simulink model "simscape1"  (R2016b)
settings: Solver=VariableStepAuto  StartTime=0.0  StopTime=3600*3  RelTol=1e-3
libraries: fl_lib x8, nesl_utility x4
settings Model: Creator=Gyulai László  LastModifiedBy=gylaszlo

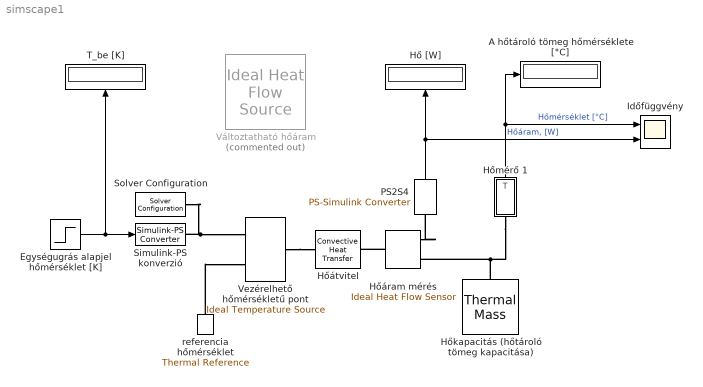
== system simscape1 ==
  A hőtároló tömeg hőmérséklete [°C] : Display
  Egységugrás alapjel hőmérséklet [K] : Step  Before=273  After=293  SampleTime=0
  Hő [W] : Display
  Hőkapacitás (hőtároló tömeg kapacitása) : fl_lib/Thermal/Thermal Elements/Thermal Mass  mass=1.5 kg  sp_heat=840 J/kg/K  T_specify=on  T_priority=High  T=0 degC  Q_specify=off  Q_priority=None  Q=0 J/s
  Hőmérő 1 : Subsystem
  Hőáram mérés : fl_lib/Thermal/Thermal Sensors/Ideal Heat Flow Sensor
  "Hőátvitel " : fl_lib/Thermal/Thermal Elements/Convective Heat Transfer  area=0.125 m^2  heat_tr_coeff=5 W/(m^2 * K)  Q_specify=off  Q_priority=None  Q=0 J/s  T_specify=off  T_priority=None  T=0 K
  Időfüggvény : Scope  NumInputPorts=2
  PS2S4 : nesl_utility/PS-Simulink Converter  PhysicalDomain=network_engine_domain  SubClassName=ps_output  LeftPortType=input  RightPortType=output  PseudoPeriodic=off  Frequencies=[]  Unit=J/s  AffineConversion=on
  Simulink-PS konverzió : nesl_utility/Simulink-PS Converter  PhysicalDomain=network_engine_domain  SubClassName=ps_input  LeftPortType=input  RightPortType=output  PseudoPeriodic=off  Frequencies=[]  NoiseDistribution=none  NoiseParameters=[]  Unit=K  AffineConversion=off  InputFiltering=off  SimscapeFilterOrder=1  InputFilterTimeConstant=0.001  UdotUserProvided=2
  Solver Configuration : nesl_utility/Solver Configuration  PhysicalDomain=network_engine_domain  SubClassName=solver  LeftPortType=input  RightPortType=generic  Accelerate=off  Tones=[]  Harmonics=[]  SimulateNoise=off  Profile=off  UseLocalSampling=off  EnableSwitchedLinearOptims=on  FrequencyDomain=off  UseCCode=off  RelTol=0.001  AbsTol=1e-06  MinStep=1e-09  ToWorkspace=off  RevertToSquareIcSolve=off  NumHomotopyIterations=100  PhasorMode=off  PhasorModeNumHarmonics=1  OverrideAbsTol=off  DoDC=off  ResidualTolerance=1e-09  UseLocalSolver=off  LocalSolverChoice=NE_BACKWARD_EULER_ADVANCER  LocalSolverSampleTime=0.001  DoFixedCost=off  MaxNonlinIter=3  MaxModeIter=2  LinearAlgebra=Sparse  DelaysMemoryBudget=1024  AutomaticFiltering=on  FilteringTimeConstant=0.001
  T_be [K] : Display
  Vezérelhető hőmérsékletű pont : fl_lib/Thermal/Thermal Sources/Ideal Temperature Source
  Változtatható hőáram : fl_lib/Thermal/Thermal Sources/Ideal Heat Flow Source  Commented=on
  referencia hőmérséklet : fl_lib/Thermal/Thermal Elements/Thermal Reference
  wires:
  Egységugrás alapjel hőmérséklet [K]/1 -> T_be [K]/1, Simulink-PS konverzió/1
  PS2S4/1 -> Hő [W]/1, Időfüggvény/2  "Hőáram, [W]"
  Hőmérő 1/1(T) -> A hőtároló tömeg hőmérséklete [°C]/1, Időfüggvény/1  "Hőmérséklet [°C]"
  connections:
  Vezérelhető hőmérsékletű pont/LConn1 -- "Hőátvitel "/LConn1
  referencia hőmérséklet/LConn1 -- Vezérelhető hőmérsékletű pont/RConn2
  Simulink-PS konverzió/RConn1 -- Solver Configuration/RConn1 -- Vezérelhető hőmérsékletű pont/RConn1
  Hőáram mérés/RConn1 -- PS2S4/LConn1
  Hőáram mérés/LConn1 -- "Hőátvitel "/RConn1
  Hőkapacitás (hőtároló tömeg kapacitása)/LConn1 -- Hőmérő 1/LConn1 -- Hőáram mérés/RConn2

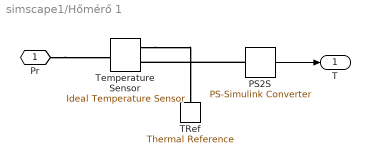
== system simscape1/Hőmérő 1 ==
  PS2S : nesl_utility/PS-Simulink Converter  PhysicalDomain=network_engine_domain  SubClassName=ps_output  LeftPortType=input  RightPortType=output  PseudoPeriodic=off  Frequencies=[]  Unit=degC  AffineConversion=on
  TRef : fl_lib/Thermal/Thermal Elements/Thermal Reference
  Temperature Sensor : fl_lib/Thermal/Thermal Sensors/Ideal Temperature Sensor
  Pr : PMIOPort  Port=1  Side=Left
  T : Outport
  wires:
  PS2S/1 -> T/1
  connections:
  Temperature Sensor/RConn1 -- TRef/LConn1
  PS2S/LConn1 -- Temperature Sensor/RConn2
  Pr/RConn1 -- Temperature Sensor/LConn1
